simulink model "model_constInput_IPC"  (R2021b)
settings: Solver=ode4  StartTime=0.0  StopTime=simOpt.SLmaxTime  FixedStep=simOpt.SLsmplTime  RelTol=1e-3
values from neighbouring files (symbols this model uses):
  simOpt = simOptTmpl    [doSingleSim.m]    (also in doSingleSimVal.m)
  SLin = struct()    [doSingleSim.m]    (also in doSingleSimVal.m)
undefined symbols (not defined in the file or in its folder): DiscIntNeverNeededParam, Parameter, rpm2radDs, strmatch
libraries: simulink x14, dspstat3 x7, cstblocks x6, slpidlib x1
settings Model: Creator=Hazim Namik  LastModifiedBy=Manuel
settings SolverCC: AlgebraicLoopSolver=LineSearch
settings DataIOCC: LimitDataPoints=on  SaveFormat=Array  SaveOutput=off  SignalLogging=off  SaveTime=off  SignalLoggingName=sigsOut
settings OptimizationCC: BlockReduction=off  BooleanDataType=off  LifeSpan=inf
settings DebuggingCC: SaveWithParameterizedLinksMsg=none  UnderspecifiedInitializationDetection=Classic  MergeDetectMultiDrivingBlocksExec=none  AllowSymbolicDim=off  PregeneratedLibrarySubsystemCodeDiagnostic=none  SFUnexpectedBacktrackingDiag=warning  SFNoUnconditionalDefaultTransitionDiag=warning  SFExecutionAtInitializationDiag=none  SFMachineParentedDataDiag=warning  ArithmeticOperatorsInVariantConditions=warning
settings HardwareCC: ProdBitPerPointer=32  ProdBitPerSizeT=32  ProdBitPerPtrDiffT=32  ProdLargestAtomicFloat=None  ProdIntDivRoundTo=Undefined  ProdEndianess=Unspecified  ProdWordSize=32  ProdHWDeviceType=32-bit Generic  TargetBitPerPointer=64  TargetBitPerSizeT=64  TargetBitPerPtrDiffT=64  TargetLongLongMode=on  TargetIntDivRoundTo=Zero  TargetEndianess=LittleEndian  TargetWordSize=64  TargetHWDeviceType=MATLAB Host  ProdEqTarget=off
settings ModelReferenceCC: PropagateSignalLabelsOutOfModel=off
settings SFSimCC: SimUseLocalCustomCode=off  CustomCodeUndefinedFunction=UseInterfaceOnly
settings RTWCC: RTWUseLocalCustomCode=off
settings CodeAppCC: StateflowObjectComments=on
settings GRTTargetCC: TargetLangStandard=C89/C90 (ANSI)
settings ConfigComp: CovMetricSettings=dw  CovSaveCumulativeToWorkspaceVar=on  CovSaveSingleToWorkspaceVar=on  CovExternalEMLEnable=off  CovSFcnEnable=off

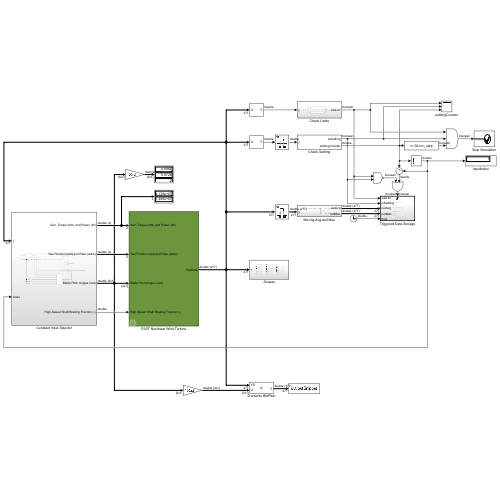
[thumbnail: Simulink's stored preview of the top-level diagram]
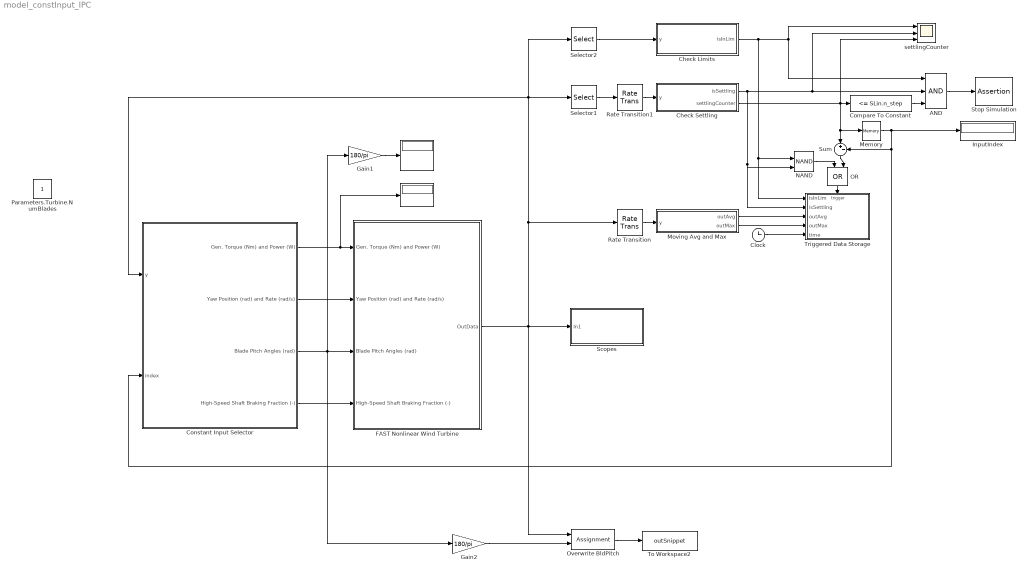
== system model_constInput_IPC ==
  " " : Display
  "  " : Display
  AND : Logic  Inputs=3  IconShape=distinctive  AllPortsSameDT=off  OutDataTypeStr=boolean
  Check Limits : Subsystem
  Check Settling : Subsystem
  Clock : Clock
  Compare To Constant : simulink/Logic and Bit Operations/Compare To Constant  relop=<=  const=SLin.n_step  OutDataTypeStr=boolean
  Constant Input Selector : Subsystem
  FAST Nonlinear Wind Turbine : Subsystem  mask(FAST Nonlinear Wind Turbine){}
      mask help: This block contains the FAST S-Function.
      mask init:
      | clear FAST_SFunc
  Gain1 : Gain  Gain=180/pi
  Gain2 : Gain  Gain=180/pi
  InputIndex : Display
  Memory : Memory  InitialCondition=1
  Moving Avg and Max : Subsystem
  NAND : Logic  Operator=NAND  IconShape=distinctive  AllPortsSameDT=off  OutDataTypeStr=boolean
  OR : Logic  Operator=OR  IconShape=distinctive  AllPortsSameDT=off  OutDataTypeStr=boolean
  Overwrite BldPitch : Assignment  DiagnosticForDimensions=Warning  IndexOptions=Index vector (dialog)  Indices=[simOpt.idx.y.BldPitch1 simOpt.idx.y.BldPitch2 simOpt.idx.y.BldPitch3]  OutputSizes=1
  Rate Transition : RateTransition
  Rate Transition1 : RateTransition
  Scopes : Subsystem
  Selector1 : Selector  InputPortWidth=simOpt.n_out  IndexOptions=Index vector (dialog)  Indices=simOpt.idx.y.settling  OutputSizes=1
  Selector2 : Selector  InputPortWidth=simOpt.n_out  IndexOptions=Index vector (dialog)  Indices=simOpt.idx.y.limCheck  OutputSizes=1
  Stop Simulation : Assertion  AssertionFailFcn=set_param(bdroot,'SimulationCommand','stop')  StopWhenAssertionFail=off
  Sum : Sum  Inputs=|+-
  To Workspace2 : ToWorkspace  VariableName=outSnippet  SampleTime=-1
      settings: MaxDataPoints=simOpt.settlingMovAvgWindowLength*5
  "Triggered Data Storage " : Subsystem  TreatAsAtomicUnit=on
  settlingCounter : Scope  NumInputPorts=3
  Parameters.Turbine.NumBlades : Constant  IOType=siggen
  wires:
  Selector1/1 -> Rate Transition1/1
  Rate Transition/1 -> Moving Avg and Max/1(y)
  Rate Transition1/1 -> Check Settling/1(y)
  Selector2/1 -> Check Limits/1(y)
  Check Limits/1(isInLim) -> NAND/1, "Triggered Data Storage "/1(isInLim), settlingCounter/1, AND/1
  Check Settling/1(isSettling) -> NAND/2, "Triggered Data Storage "/2(isSettling), settlingCounter/2, AND/2
  Moving Avg and Max/1(outAvg) -> "Triggered Data Storage "/3(outAvg)
  AND/1 -> Stop Simulation/1
  Compare To Constant/1 -> AND/3
  Clock/1 -> "Triggered Data Storage "/5(time)
  Check Settling/2(settlingCounter) -> Sum/1, Memory/1, settlingCounter/3, Compare To Constant/1
  Memory/1 -> InputIndex/1, Constant Input Selector/2(index), Sum/2
  Constant Input Selector/1(Gen. Torque (Nm) and Power (W)) -> "  "/1, FAST Nonlinear Wind Turbine/1(Gen. Torque (Nm) and Power (W))
  Constant Input Selector/2(Yaw Position (rad) and Rate (rad/s)) -> FAST Nonlinear Wind Turbine/2(Yaw Position (rad) and Rate (rad/s))
  Constant Input Selector/3(Blade Pitch Angles (rad)) -> Gain2/1, Gain1/1, FAST Nonlinear Wind Turbine/3(Blade Pitch Angles (rad))
  Constant Input Selector/4(High-Speed Shaft Braking Fraction (-)) -> FAST Nonlinear Wind Turbine/4(High-Speed Shaft Braking Fraction (-))
  Gain1/1 -> " "/1
  OR/1 -> "Triggered Data Storage "/Trigger
  Sum/1 -> OR/2
  NAND/1 -> OR/1
  FAST Nonlinear Wind Turbine/1(OutData) -> Overwrite BldPitch/1, Constant Input Selector/1(y), Selector1/1, Selector2/1, Rate Transition/1, Scopes/1(In1)
  Moving Avg and Max/2(outMax) -> "Triggered Data Storage "/4(outMax)
  Overwrite BldPitch/1 -> To Workspace2/1
  Gain2/1 -> Overwrite BldPitch/2

== system model_constInput_IPC/Check Limits ==
  y : Inport
  Compare To Constant : simulink/Logic and Bit Operations/Compare To Constant  relop=<=  const=simOpt.limCheckLowerBound  OutDataTypeStr=boolean
  Compare To Constant1 : simulink/Logic and Bit Operations/Compare To Constant  relop=>=  const=simOpt.limCheckUpperBound  OutDataTypeStr=boolean
  OR : Logic  Operator=NOR  IconShape=distinctive  AllPortsSameDT=off  OutDataTypeStr=boolean
  isInLim : Outport
  wires:
  y/1 -> Compare To Constant1/1, Compare To Constant/1
  OR/1 -> isInLim/1
  Compare To Constant1/1 -> OR/2
  Compare To Constant/1 -> OR/1

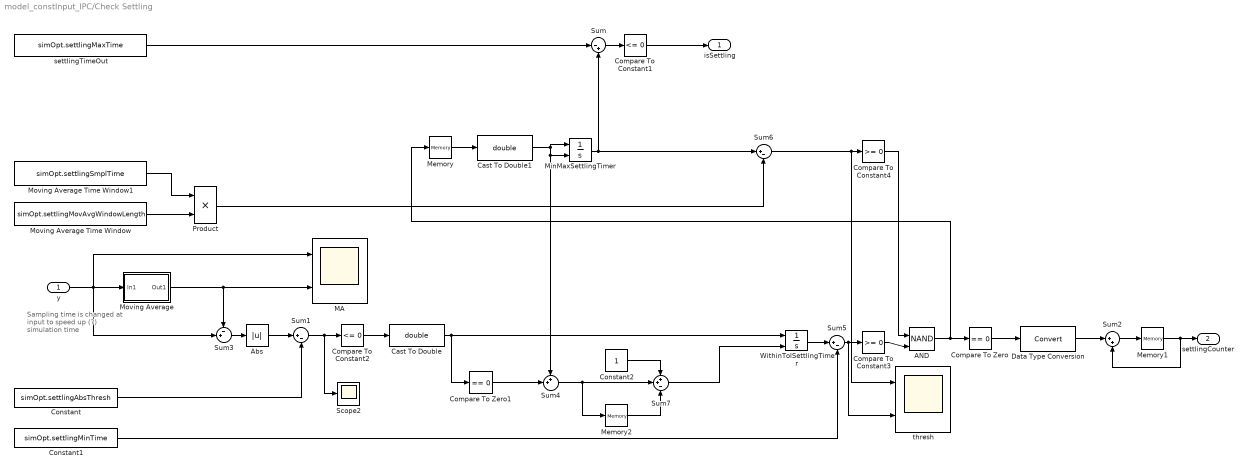
== system model_constInput_IPC/Check Settling ==
  note: Sampling time is changed at input
      | to speed up (?) simulation time
  y : Inport  SampleTime=simOpt.settlingSmplTime
  AND : Logic  Operator=NAND  IconShape=distinctive  AllPortsSameDT=off  OutDataTypeStr=boolean
  Abs : Abs
  Cast To Double : DataTypeConversion  OutDataTypeStr=double
  Cast To Double1 : DataTypeConversion  OutDataTypeStr=double
  Compare To Constant1 : simulink/Logic and Bit Operations/Compare To Constant  relop=<=  const=0  OutDataTypeStr=boolean
  Compare To Constant2 : simulink/Logic and Bit Operations/Compare To Constant  relop=<=  const=0  OutDataTypeStr=boolean
  Compare To Constant3 : simulink/Logic and Bit Operations/Compare To Constant  relop=>=  const=0  OutDataTypeStr=boolean
  Compare To Constant4 : simulink/Logic and Bit Operations/Compare To Constant  relop=>=  const=0  OutDataTypeStr=boolean
  Compare To Zero : simulink/Logic and Bit Operations/Compare To Zero  relop===  OutDataTypeStr=boolean
  Compare To Zero1 : simulink/Logic and Bit Operations/Compare To Zero  relop===  OutDataTypeStr=boolean
  Constant : Constant  Value=simOpt.settlingAbsThresh
  Constant1 : Constant  Value=simOpt.settlingMinTime
  Constant2 : Constant
  Data Type Conversion : DataTypeConversion
  MA : Scope  NumInputPorts=2
  Memory : Memory  InitialCondition=true
  Memory1 : Memory  InitialCondition=1  InheritSampleTime=on
  Memory2 : Memory  InitialCondition=1  InheritSampleTime=on
  MinMaxSettlingTimer : Integrator  ExternalReset=falling  LimitOutput=on  UpperSaturationLimit=max(simOpt.settlingMovAvgWindowLength*simOpt.settlingSmplTime,simOpt.settlingMaxTime)*1.01
  Moving Average : Subsystem
  Moving Average Time Window : Constant  Value=simOpt.settlingMovAvgWindowLength
  Moving Average Time Window1 : Constant  Value=simOpt.settlingSmplTime
  Product : Product
  Scope2 : Scope
  Sum : Sum  Inputs=|-+
  Sum1 : Sum  Inputs=|+-
  Sum2 : Sum  Inputs=|++
  Sum3 : Sum  Inputs=-+|
  Sum4 : Sum  Inputs=++|
  Sum5 : Sum  Inputs=|+-
  Sum6 : Sum  Inputs=|+-
  Sum7 : Sum  Inputs=++-
  WithinTolSettlingTimer : Integrator  ExternalReset=falling  LimitOutput=on  UpperSaturationLimit=simOpt.settlingMinTime
  settlingTimeOut : Constant  Value=simOpt.settlingMaxTime
  thresh : Scope  NumInputPorts=2
  isSettling : Outport
  settlingCounter : Outport  Port=2
  wires:
  AND/1 -> Compare To Zero/1, Memory/1
  MinMaxSettlingTimer/1 -> Sum6/1, Sum/2
  Sum6/1 -> thresh/1, Compare To Constant4/1
  Sum1/1 -> Scope2/1, Compare To Constant2/1
  WithinTolSettlingTimer/1 -> Sum5/1
  y/1 -> MA/1, Moving Average/1(In1), Sum3/2
  Abs/1 -> Sum1/1
  Sum3/1 -> Abs/1
  Sum5/1 -> thresh/2, Compare To Constant3/1
  Moving Average Time Window/1 -> Product/2
  Compare To Constant2/1 -> Cast To Double/1
  Constant/1 -> Sum1/2
  Constant1/1 -> Sum5/2
  Compare To Constant3/1 -> AND/2
  Compare To Constant4/1 -> AND/1
  Memory/1 -> Cast To Double1/1
  Cast To Double1/1 -> Sum4/1, MinMaxSettlingTimer/2, MinMaxSettlingTimer/1
  Moving Average/1(Out1) -> Sum3/1, MA/2
  settlingTimeOut/1 -> Sum/1
  Sum/1 -> Compare To Constant1/1
  Compare To Constant1/1 -> isSettling/1
  Memory1/1 -> settlingCounter/1, Sum2/2
  Sum2/1 -> Memory1/1
  Compare To Zero/1 -> Data Type Conversion/1
  Data Type Conversion/1 -> Sum2/1
  Moving Average Time Window1/1 -> Product/1
  Product/1 -> Sum6/2
  Sum7/1 -> WithinTolSettlingTimer/2
  Compare To Zero1/1 -> Sum4/2
  Cast To Double/1 -> WithinTolSettlingTimer/1, Compare To Zero1/1
  Sum4/1 -> Sum7/2, Memory2/1
  Memory2/1 -> Sum7/3
  Constant2/1 -> Sum7/1

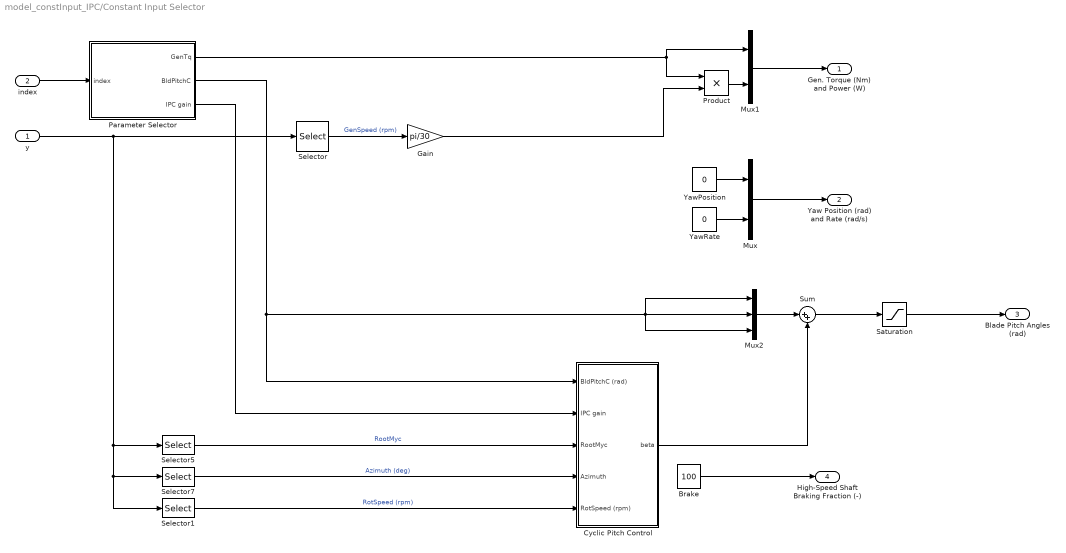
== system model_constInput_IPC/Constant Input Selector ==
  y : Inport
  index : Inport  Port=2
  Brake : Constant  Value=100
  Cyclic Pitch Control : Subsystem
  Gain : Gain  Gain=pi/30
  Mux : Mux  Inputs=2
  Mux1 : Mux  Inputs=2
  Mux2 : Mux  Inputs=3
  Parameter Selector : Subsystem
  Product : Product
  Saturation : Saturate  UpperLimit=inf  LowerLimit=deg2rad(simOpt.BldPitch_min)
  Selector : Selector  InputPortWidth=simOpt.n_out  IndexOptions=Index vector (dialog)  Indices=simOpt.idx.y.GenSpeed  OutputSizes=1
  Selector1 : Selector  InputPortWidth=simOpt.n_out  IndexOptions=Index vector (dialog)  Indices=simOpt.idx.y.RotSpeed  OutputSizes=1
  Selector5 : Selector  InputPortWidth=simOpt.n_out  IndexOptions=Index vector (dialog)  Indices=[simOpt.idx.y.RootMyc1 simOpt.idx.y.RootMyc2 simOpt.idx.y.RootMyc3]  OutputSizes=1
  Selector7 : Selector  InputPortWidth=simOpt.n_out  IndexOptions=Index vector (dialog)  Indices=simOpt.idx.y.Azimuth  OutputSizes=1
  Sum : Sum  Inputs=|++
  YawPosition : Constant  Value=0
  YawRate : Constant  Value=0
  Gen. Torque (Nm) and Power (W) : Outport
  Yaw Position (rad) and Rate (rad/s) : Outport  Port=2
  Blade Pitch Angles (rad) : Outport  Port=3
  High-Speed Shaft Braking Fraction (-) : Outport  Port=4
  wires:
  YawRate/1 -> Mux/2
  index/1 -> Parameter Selector/1(index)
  YawPosition/1 -> Mux/1
  Product/1 -> Mux1/2
  Brake/1 -> High-Speed Shaft Braking Fraction (-)/1
  Mux1/1 -> Gen. Torque (Nm) and Power (W)/1
  Mux/1 -> Yaw Position (rad) and Rate (rad/s)/1
  Gain/1 -> Product/2
  Parameter Selector/2(BldPitchC) -> Cyclic Pitch Control/1(BldPitchC (rad)), Mux2/1, Mux2/3, Mux2/2
  Mux2/1 -> Sum/1
  y/1 -> Selector/1, Selector1/1, Selector7/1, Selector5/1
  Selector/1 -> Gain/1  "GenSpeed (rpm)"
  Selector5/1 -> Cyclic Pitch Control/3(RootMyc)  "RootMyc"
  Selector7/1 -> Cyclic Pitch Control/4(Azimuth)  "Azimuth (deg)"
  Cyclic Pitch Control/1(beta) -> Sum/2
  Parameter Selector/3(IPC gain) -> Cyclic Pitch Control/2(IPC gain)
  Parameter Selector/1(GenTq) -> Mux1/1, Product/1
  Selector1/1 -> Cyclic Pitch Control/5(RotSpeed (rpm))  "RotSpeed (rpm)"
  Sum/1 -> Saturation/1
  Saturation/1 -> Blade Pitch Angles (rad)/1

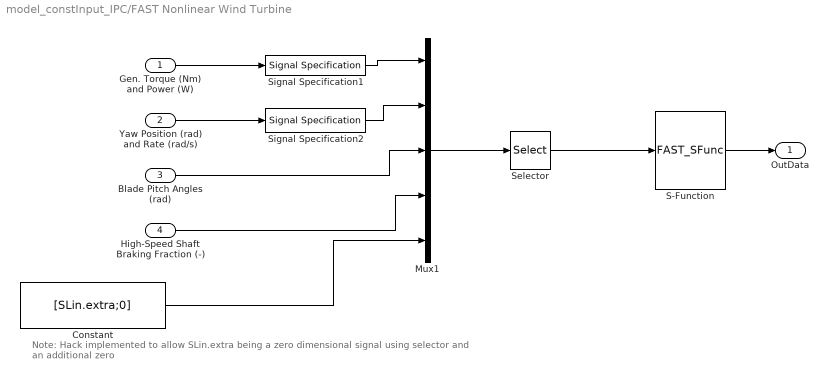
== system model_constInput_IPC/FAST Nonlinear Wind Turbine ==
  note: Note: Hack implemented to allow SLin.extra being a zero dimensional signal using selector and an additional zero
  Gen. Torque (Nm) and Power (W) : Inport
  Yaw Position (rad) and Rate (rad/s) : Inport  Port=2
  Blade Pitch Angles (rad) : Inport  Port=3
  High-Speed Shaft Braking Fraction (-) : Inport  Port=4
  Constant : Constant  Value=[SLin.extra;0]
  Mux1 : Mux  Inputs=5
  S-Function : S-Function  FunctionName=FAST_SFunc  Parameters=simOpt.FSTnewInputFile, simOpt.SLmaxTime, 0  SFunctionDeploymentMode=off  EnableBusSupport=off
  Selector : Selector  InputPortWidth=9+numel(SLin.extra)  IndexOptions=Index vector (dialog)  Indices=1:(8+numel(SLin.extra))  OutputSizes=1
  Signal Specification1 : SignalSpecification  OutDataTypeStr=double  Dimensions=2
  Signal Specification2 : SignalSpecification  OutDataTypeStr=double  Dimensions=2
  OutData : Outport  VectorParamsAs1DForOutWhenUnconnected=off
  wires:
  Gen. Torque (Nm) and Power (W)/1 -> Signal Specification1/1
  S-Function/1 -> OutData/1
  Mux1/1 -> Selector/1
  Blade Pitch Angles (rad)/1 -> Mux1/3
  Yaw Position (rad) and Rate (rad/s)/1 -> Signal Specification2/1
  Signal Specification1/1 -> Mux1/1
  Signal Specification2/1 -> Mux1/2
  High-Speed Shaft Braking Fraction (-)/1 -> Mux1/4
  Constant/1 -> Mux1/5
  Selector/1 -> S-Function/1

== system model_constInput_IPC/Moving Avg and Max ==
  note: Sampling time is changed at input
      | to speed up (?) simulation time
  y : Inport  SampleTime=simOpt.settlingSmplTime
  Moving Maximum : dspstat3/Moving Maximum  SpecifyWindowLength=on  WindowLength=simOpt.settlingMovAvgWindowLength  SimulateUsing=Interpreted execution
      settings: SourceProductBaseCode=DS
  Moving Average : dspstat3/Moving Average  Method=Sliding window  ForgettingFactorPort=off  SpecifyWindowLength=on  WindowLength=simOpt.settlingMovAvgWindowLength  ForgettingFactor=0.99  SimulateUsing=Interpreted execution
  Reshape : Reshape  OutputDimensionality=Row vector (2-D)
  Reshape1 : Reshape
  Reshape2 : Reshape
  outAvg : Outport
  outMax : Outport  Port=2
  wires:
  y/1 -> Reshape/1
  Moving Average/1 -> Reshape1/1
  Reshape/1 -> Moving Maximum/1, Moving Average/1
  Reshape1/1 -> outAvg/1
  Reshape2/1 -> outMax/1
  Moving Maximum/1 -> Reshape2/1

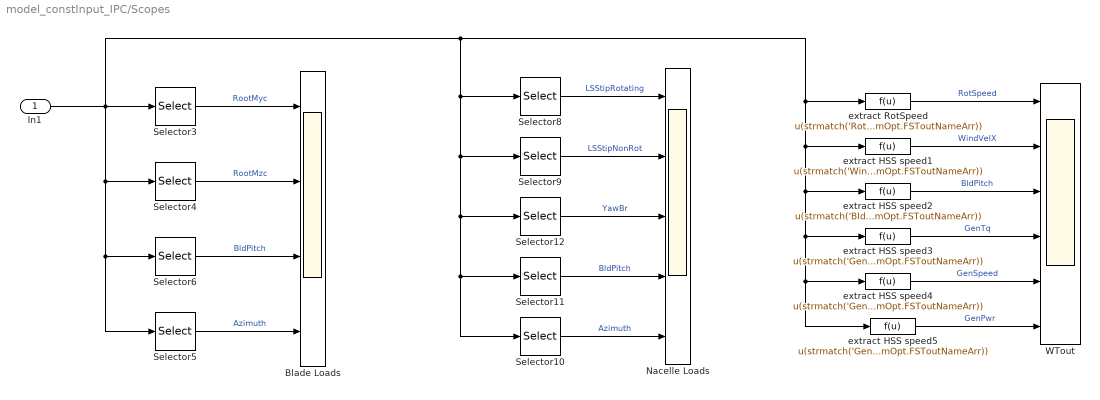
== system model_constInput_IPC/Scopes ==
  In1 : Inport
  Blade Loads : Scope  NumInputPorts=4
  Nacelle Loads : Scope  NumInputPorts=5
  Selector10 : Selector  InputPortWidth=simOpt.n_out  IndexOptions=Index vector (dialog)  Indices=[simOpt.idx.y.Azimuth]  OutputSizes=1
  Selector11 : Selector  InputPortWidth=simOpt.n_out  IndexOptions=Index vector (dialog)  Indices=[simOpt.idx.y.BldPitch1 simOpt.idx.y.BldPitch2 simOpt.idx.y.BldPitch3]  OutputSizes=1
  Selector12 : Selector  InputPortWidth=simOpt.n_out  IndexOptions=Index vector (dialog)  Indices=[simOpt.idx.y.YawBrMyp simOpt.idx.y.YawBrMzp]  OutputSizes=1
  Selector3 : Selector  InputPortWidth=simOpt.n_out  IndexOptions=Index vector (dialog)  Indices=[simOpt.idx.y.RootMyc1 simOpt.idx.y.RootMyc2 simOpt.idx.y.RootMyc3]  OutputSizes=1
  Selector4 : Selector  InputPortWidth=simOpt.n_out  IndexOptions=Index vector (dialog)  Indices=[simOpt.idx.y.RootMzc1 simOpt.idx.y.RootMzc2 simOpt.idx.y.RootMzc3]  OutputSizes=1
  Selector5 : Selector  InputPortWidth=simOpt.n_out  IndexOptions=Index vector (dialog)  Indices=[simOpt.idx.y.Azimuth]  OutputSizes=1
  Selector6 : Selector  InputPortWidth=simOpt.n_out  IndexOptions=Index vector (dialog)  Indices=[simOpt.idx.y.BldPitch1 simOpt.idx.y.BldPitch2 simOpt.idx.y.BldPitch3]  OutputSizes=1
  Selector8 : Selector  InputPortWidth=simOpt.n_out  IndexOptions=Index vector (dialog)  Indices=[simOpt.idx.y.LSSTipMya simOpt.idx.y.LSSTipMza]  OutputSizes=1
  Selector9 : Selector  InputPortWidth=simOpt.n_out  IndexOptions=Index vector (dialog)  Indices=[simOpt.idx.y.LSSTipMys simOpt.idx.y.LSSTipMzs]  OutputSizes=1
  WTout : Scope  NumInputPorts=6
  extract HSS speed1 : Fcn  Expr=u(strmatch('Wind1VelX',simOpt.FSToutNameArr))
  extract HSS speed2 : Fcn  Expr=u(strmatch('BldPitch1',simOpt.FSToutNameArr))
  extract HSS speed3 : Fcn  Expr=u(strmatch('GenTq',simOpt.FSToutNameArr))
  extract HSS speed4 : Fcn  Expr=u(strmatch('GenSpeed',simOpt.FSToutNameArr))
  extract HSS speed5 : Fcn  Expr=u(strmatch('GenPwr',simOpt.FSToutNameArr))
  extract RotSpeed : Fcn  Expr=u(strmatch('RotSpeed',simOpt.FSToutNameArr))
  wires:
  In1/1 -> Selector5/1, Selector6/1, Selector4/1, Selector10/1, Selector11/1, Selector12/1, Selector9/1, Selector8/1, extract RotSpeed/1, extract HSS speed1/1, extract HSS speed3/1, extract HSS speed4/1, extract HSS speed5/1, extract HSS speed2/1, Selector3/1
  Selector6/1 -> Blade Loads/3  "BldPitch"
  Selector9/1 -> Nacelle Loads/2  "LSStipNonRot"
  extract HSS speed5/1 -> WTout/6  "GenPwr"
  Selector3/1 -> Blade Loads/1  "RootMyc"
  Selector8/1 -> Nacelle Loads/1  "LSStipRotating"
  Selector11/1 -> Nacelle Loads/4  "BldPitch"
  extract HSS speed2/1 -> WTout/3  "BldPitch"
  extract RotSpeed/1 -> WTout/1  "RotSpeed"
  Selector5/1 -> Blade Loads/4  "Azimuth"
  Selector12/1 -> Nacelle Loads/3  "YawBr"
  extract HSS speed4/1 -> WTout/5  "GenSpeed"
  extract HSS speed1/1 -> WTout/2  "WindVelX"
  Selector10/1 -> Nacelle Loads/5  "Azimuth"
  extract HSS speed3/1 -> WTout/4  "GenTq"
  Selector4/1 -> Blade Loads/2  "RootMzc"

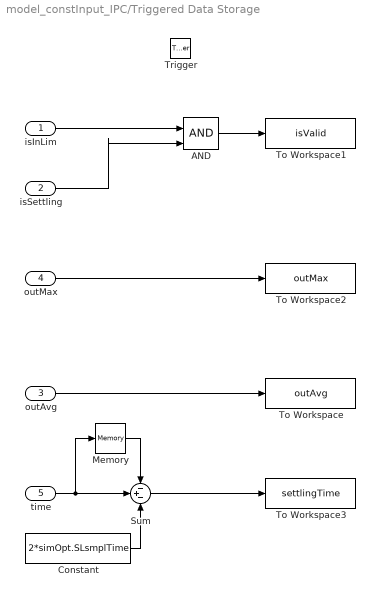
== system model_constInput_IPC/Triggered Data Storage  ==
  isInLim : Inport
  isSettling : Inport  Port=2
  outAvg : Inport  Port=3
  outMax : Inport  Port=4
  time : Inport  Port=5
  Trigger : TriggerPort  VariantControl=(inherit)
  AND : Logic  IconShape=distinctive  AllPortsSameDT=off  OutDataTypeStr=boolean
  Constant : Constant  Value=2*simOpt.SLsmplTime
  Memory : Memory  InheritSampleTime=on
  Sum : Sum  Inputs=-+-
  To Workspace : ToWorkspace  VariableName=outAvg  SampleTime=-1
  To Workspace1 : ToWorkspace  VariableName=isValid  SampleTime=-1
  To Workspace2 : ToWorkspace  VariableName=outMax  SampleTime=-1
  To Workspace3 : ToWorkspace  VariableName=settlingTime  SampleTime=-1
  wires:
  outAvg/1 -> To Workspace/1
  isInLim/1 -> AND/1
  isSettling/1 -> AND/2
  Sum/1 -> To Workspace3/1
  time/1 -> Sum/2, Memory/1
  AND/1 -> To Workspace1/1
  Constant/1 -> Sum/3
  Memory/1 -> Sum/1
  outMax/1 -> To Workspace2/1

== system model_constInput_IPC/Check Settling/Moving Average ==
  In1 : Inport
  Moving Average : dspstat3/Moving Average  Method=Sliding window  ForgettingFactorPort=off  SpecifyWindowLength=on  WindowLength=simOpt.settlingMovAvgWindowLength  ForgettingFactor=0.99  SimulateUsing=Interpreted execution
  Reshape : Reshape  OutputDimensionality=Row vector (2-D)
  Reshape1 : Reshape
  Out1 : Outport
  wires:
  Moving Average/1 -> Reshape1/1
  Reshape1/1 -> Out1/1
  Reshape/1 -> Moving Average/1
  In1/1 -> Reshape/1

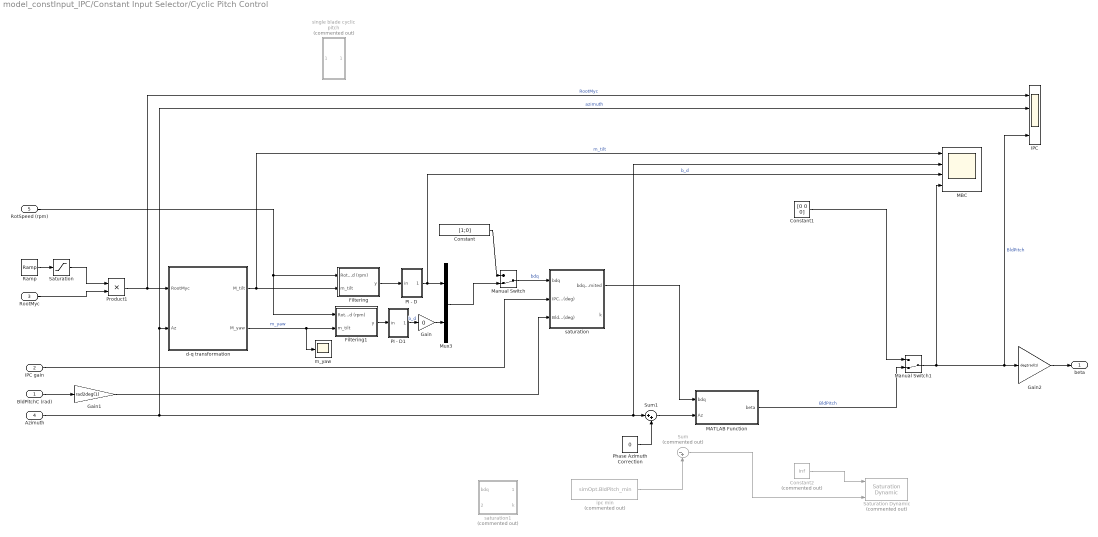
== system model_constInput_IPC/Constant Input Selector/Cyclic Pitch Control ==
  BldPitchC (rad) : Inport
  IPC gain : Inport  Port=2
  RootMyc : Inport  Port=3
  Azimuth : Inport  Port=4
  RotSpeed (rpm) : Inport  Port=5
  Constant : Constant  Value=[1;0]
  Constant1 : Constant  Value=[0 0 0]
  Constant2 : Constant  Commented=on  Value=inf
  Filtering : Subsystem
  Filtering1 : Subsystem
  Gain : Gain  Gain=0
  Gain1 : Gain  Gain=rad2deg(1)
  Gain2 : Gain  Gain=deg2rad(1)
  IPC : Scope  NumInputPorts=4
  MATLAB Function : MATLAB Function  TreatAsAtomicUnit=on
  MBC : Scope  NumInputPorts=4
  Manual Switch : ManualSwitch  CurrentSetting=0
  Manual Switch1 : ManualSwitch  CurrentSetting=0
  Mux3 : Mux  Inputs=2
  PI - D : Subsystem
  PI - D1 : Subsystem
  Phase Azimuth Correction : Constant  Value=0
  Product1 : Product
  Ramp : simulink/Sources/Ramp  slope=1  start=0  InitialOutput=0
  Saturation : Saturate  UpperLimit=1  LowerLimit=0
  Saturation Dynamic : simulink/Discontinuities/Saturation Dynamic  Commented=on  OutMin=[]  OutMax=[]  OutDataTypeStr=Inherit: Same as second input  OutDataType=fixdt(1, 16)  OutScaling=2^-10  DoSatur=off
  Sum : Sum  Commented=on  Inputs=|-+
  Sum1 : Sum  Inputs=|++
  d-q transformation : MATLAB Function  TreatAsAtomicUnit=on
  ipc min : Constant  Commented=on  Value=simOpt.BldPitch_min
  m_yaw : Scope
  saturation : Subsystem
  saturation1 : Subsystem  Commented=on
  single blade cyclic pitch : Subsystem  Commented=on
  beta : Outport
  wires:
  Azimuth/1 -> IPC/2, d-q transformation/2(Az), MBC/2, Sum1/1  "azimuth"
  d-q transformation/2(M_yaw) -> Filtering1/2(m_tilt), m_yaw/1  "m_yaw"
  Product1/1 -> IPC/1, d-q transformation/1(RootMyc)  "RootMyc"
  Filtering1/1(y) -> PI - D1/1(in)
  Constant/1 -> Manual Switch/1
  d-q transformation/1(M_tilt) -> Filtering/2(m_tilt), MBC/1  "m_tilt"
  Mux3/1 -> Manual Switch/2
  Manual Switch1/1 -> Gain2/1, IPC/4, MBC/4  "BldPitch"
  Constant1/1 -> Manual Switch1/1
  IPC gain/1 -> saturation/2(IPCbldPitch_abs_max (deg))
  Manual Switch/1 -> saturation/1(bdq)  "bdq"
  Filtering/1(y) -> PI - D/1(in)
  RotSpeed (rpm)/1 -> Filtering1/1(RotSpeed (rpm)), Filtering/1(RotSpeed (rpm))
  PI - D/1(out) -> MBC/3, Mux3/1  "b_d"
  Sum1/1 -> MATLAB Function/2(Az)
  Phase Azimuth Correction/1 -> Sum1/2
  PI - D1/1(out) -> Gain/1  "b_d"
  Gain/1 -> Mux3/2
  RootMyc/1 -> Product1/2
  Saturation/1 -> Product1/1
  Ramp/1 -> Saturation/1
  saturation/1(bdq_limited) -> MATLAB Function/1(bdq)
  BldPitchC (rad)/1 -> Gain1/1
  Gain1/1 -> saturation/3(BldPitchC (deg))
  MATLAB Function/1(beta) -> Manual Switch1/2  "BldPitch"
  ipc min/1 -> Sum/2
  Sum/1 -> Saturation Dynamic/3
  Constant2/1 -> Saturation Dynamic/1
  Gain2/1 -> beta/1

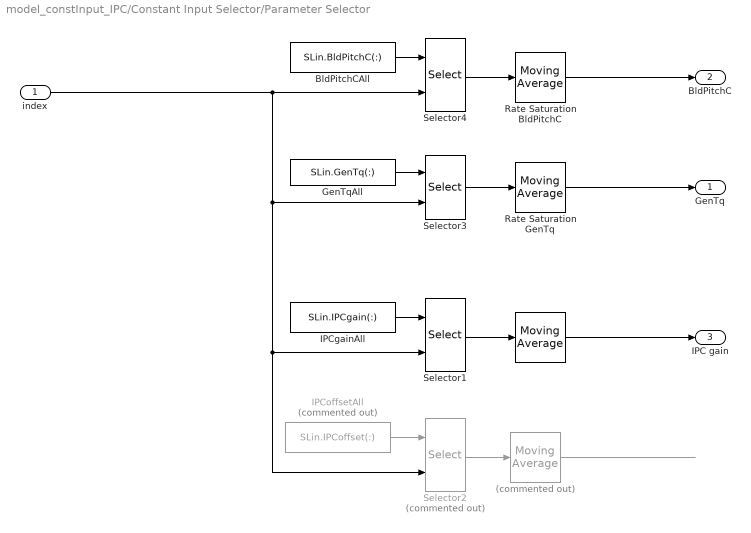
== system model_constInput_IPC/Constant Input Selector/Parameter Selector ==
  index : Inport
  " " : dspstat3/Moving Average  Method=Sliding window  ForgettingFactorPort=off  SpecifyWindowLength=on  WindowLength=8  ForgettingFactor=0.99  SimulateUsing=Interpreted execution
  "  " : dspstat3/Moving Average  Commented=on  Method=Sliding window  ForgettingFactorPort=off  SpecifyWindowLength=on  WindowLength=8  ForgettingFactor=0.99  SimulateUsing=Interpreted execution
  BldPitchCAll : Constant  Value=SLin.BldPitchC(:)
  GenTqAll : Constant  Value=SLin.GenTq(:)
  IPCgainAll : Constant  Value=SLin.IPCgain(:)
  IPCoffsetAll : Constant  Commented=on  Value=SLin.IPCoffset(:)
  Rate Saturation BldPitchC : dspstat3/Moving Average  Method=Sliding window  ForgettingFactorPort=off  SpecifyWindowLength=on  WindowLength=8  ForgettingFactor=0.99  SimulateUsing=Interpreted execution
  Rate Saturation GenTq : dspstat3/Moving Average  Method=Sliding window  ForgettingFactorPort=off  SpecifyWindowLength=on  WindowLength=8  ForgettingFactor=0.99  SimulateUsing=Interpreted execution
  Selector1 : Selector  InputPortWidth=SLin.n_step  IndexOptions=Index vector (port)  Indices=simOpt.i_outRotSpeed  OutputSizes=1
  Selector2 : Selector  Commented=on  InputPortWidth=SLin.n_step  IndexOptions=Index vector (port)  Indices=simOpt.i_outRotSpeed  OutputSizes=1
  Selector3 : Selector  InputPortWidth=SLin.n_step  IndexOptions=Index vector (port)  Indices=simOpt.i_outRotSpeed  OutputSizes=1
  Selector4 : Selector  InputPortWidth=SLin.n_step  IndexOptions=Index vector (port)  Indices=simOpt.i_outRotSpeed  OutputSizes=1
  GenTq : Outport
  BldPitchC : Outport  Port=2
  IPC gain : Outport  Port=3
  wires:
  IPCgainAll/1 -> Selector1/1
  "  "/1 -> ?
  Selector1/1 -> " "/1
  " "/1 -> IPC gain/1
  Selector2/1 -> "  "/1
  IPCoffsetAll/1 -> Selector2/1
  GenTqAll/1 -> Selector3/1
  Selector3/1 -> Rate Saturation GenTq/1
  Rate Saturation GenTq/1 -> GenTq/1
  index/1 -> Selector3/2, Selector2/2, Selector1/2, Selector4/2
  BldPitchCAll/1 -> Selector4/1
  Selector4/1 -> Rate Saturation BldPitchC/1
  Rate Saturation BldPitchC/1 -> BldPitchC/1

== system model_constInput_IPC/Constant Input Selector/Cyclic Pitch Control/Filtering ==
  RotSpeed (rpm) : Inport
  m_tilt : Inport  Port=2
  Gain1 : Gain  Gain=rpm2radDs
  Moving 3P Notch : Subsystem
  Moving 6P Notch : Subsystem  Commented=on
  Moving Low Pass : Subsystem
  y : Outport
  wires:
  Moving 3P Notch/1(y) -> Moving Low Pass/1(u)
  Gain1/1 -> Moving Low Pass/2(RotSpeed (rad/s)), Moving 3P Notch/2(RotSpeed (rad/s))
  m_tilt/1 -> Moving 3P Notch/1(u)
  RotSpeed (rpm)/1 -> Gain1/1
  Moving Low Pass/1(y) -> y/1

== system model_constInput_IPC/Constant Input Selector/Cyclic Pitch Control/Filtering1 ==
  RotSpeed (rpm) : Inport
  m_tilt : Inport  Port=2
  Gain1 : Gain  Gain=rpm2radDs
  Moving 3P Notch : Subsystem
  Moving 6P Notch : Subsystem  Commented=on
  Moving Low Pass : Subsystem
  y : Outport
  wires:
  Moving 3P Notch/1(y) -> Moving Low Pass/1(u)
  Gain1/1 -> Moving Low Pass/2(RotSpeed (rad/s)), Moving 3P Notch/2(RotSpeed (rad/s))
  m_tilt/1 -> Moving 3P Notch/1(u)
  RotSpeed (rpm)/1 -> Gain1/1
  Moving Low Pass/1(y) -> y/1

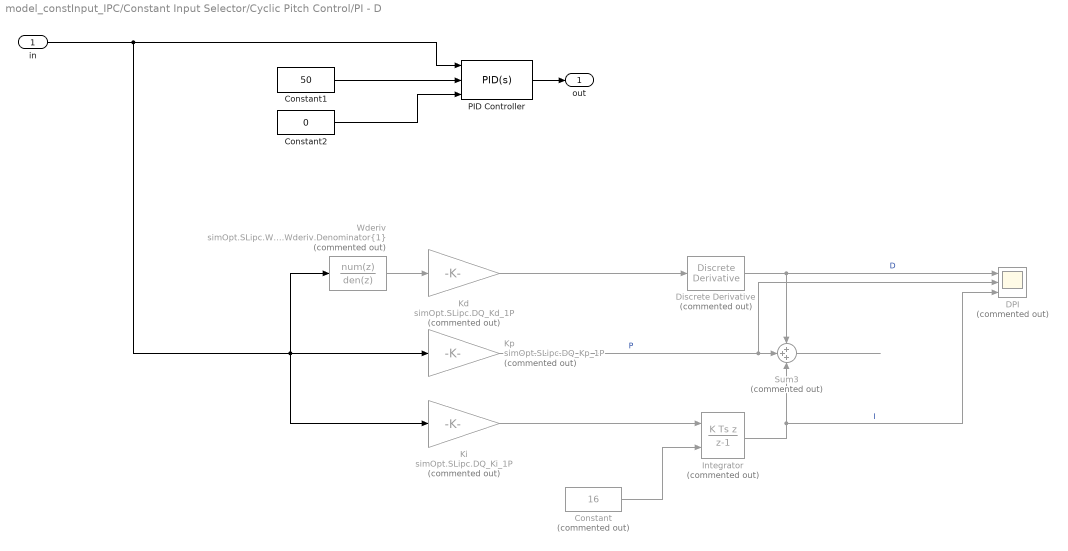
== system model_constInput_IPC/Constant Input Selector/Cyclic Pitch Control/PI - D ==
  in : Inport
  Constant : Constant  Commented=on  Value=16
  Constant1 : Constant  Value=50
  Constant2 : Constant  Value=0
  DPI : Scope  Commented=on  NumInputPorts=3
  Discrete Derivative : simulink/Discrete/Discrete Derivative  Commented=on  gainval=1.0  ICPrevScaledInput=0.0  OutMin=[]  OutMax=[]  OutDataType=fixdt(1, 16)  OutScaling=2^-10  DoSatur=off
  Integrator : DiscreteIntegrator  Commented=on  IntegratorMethod=Integration: Backward Euler  gainval=1  InitialConditionSource=external  SampleTime=-1  UpperSaturationLimit=1.570796/(.008068634/9.5492966)/(1./(1.+pi/2/.109997))  LowerSaturationLimit=0  ICPrevOutput=DiscIntNeverNeededParam  ICPrevScaledInput=DiscIntNeverNeededParam
  Kd : Gain  Commented=on  Gain=simOpt.SLipc.DQ_Kd_1P
  Ki : Gain  Commented=on  Gain=simOpt.SLipc.DQ_Ki_1P
  Kp : Gain  Commented=on  Gain=simOpt.SLipc.DQ_Kp_1P
  PID Controller : slpidlib/PID Controller  Controller=PID  Form=Parallel  TimeDomain=Continuous-time  UseExternalTs=off  SampleTime=-1  IntegratorMethod=Forward Euler  FilterMethod=Forward Euler  ControllerParametersSource=internal  P=simOpt.SLipc.DQ_Kp_1P  I=simOpt.SLipc.DQ_Ki_1P  D=simOpt.SLipc.DQ_Kd_1P  UseFilter=on  N=100  TunerSelectOption=Transfer Function Based (PID Tuner App)  InitialConditionSource=external  InitialConditionForIntegrator=0  InitialConditionForFilter=0  DifferentiatorICPrevScaledInput=0  ExternalReset=none  TrackingMode=off  Kt=1  LimitOutput=on  SatLimitsSource=internal  UpperSaturationLimit=90  LowerSaturationLimit=90  LinearizeAsGain=on  AntiWindupMode=clamping  Kb=1  POutMin=[]  POutMax=[]  IOutMin=[]  IOutMax=[]  DOutMin=[]  DOutMax=[]  NOutMin=[]  NOutMax=[]  SumOutMin=[]  SumOutMax=[]  SaturationOutMin=[]  SaturationOutMax=[]  PParamMin=[]  PParamMax=[]  IParamMin=[]  IParamMax=[]  DParamMin=[]  DParamMax=[]  NParamMin=[]  NParamMax=[]  KbParamMin=[]  KbParamMax=[]  KtParamMin=[]  KtParamMax=[]  KbOutMin=[]  KbOutMax=[]  KtOutMin=[]  KtOutMax=[]  IntegratorOutMin=[]  IntegratorOutMax=[]  FilterOutMin=[]  FilterOutMax=[]  SumI1OutMin=[]  SumI1OutMax=[]  SumI2OutMin=[]  SumI2OutMax=[]  SumI3OutMin=[]  SumI3OutMax=[]  SumI4OutMin=[]  SumI4OutMax=[]  SumDOutMin=[]  SumDOutMax=[]  DifferentiatorOutMin=[]  DifferentiatorOutMax=[]  FilterDiffOutCoefMin=[]  FilterDiffOutCoefMax=[]  ReciprocalOutMin=[]  ReciprocalOutMax=[]  SumDenOutMin=[]  SumDenOutMax=[]  SumNumOutMin=[]  SumNumOutMax=[]  DivideOutMin=[]  DivideOutMax=[]  UdiffTsProdOutMin=[]  UdiffTsProdOutMax=[]  NTsProdOutMin=[]  NTsProdOutMax=[]  UintegralTsProdOutMin=[]  UintegralTsProdOutMax=[]  UngainTsProdOutMin=[]  UngainTsProdOutMax=[]  IntegratorContinuousStateAttributes=''  IntegratorStateMustResolveToSignalObject=off  IntegratorRTWStateStorageClass=Auto  FilterContinuousStateAttributes=''  FilterStateMustResolveToSignalObject=off  FilterRTWStateStorageClass=Auto  ParallelPVariant=InternalParameters  IdealPVariant=Disabled  IVariant=InternalParameters  DVariant=InternalParameters  IntegratorVariant=Continuous  SatVariant=Enabled  AWVariant=ContClampingParallel  PCopyVariant=Disabled  TRVariant=Disabled  FdbkBlocksVariant=Forward  IdealPFdbkVariant=Disabled  SatFdbkVariant=Disabled  DerivativeFilterVariant=ContFilter  NVariant=InternalParameters  NCopyVariant=Disabled  FilterICVariant=ExternalICs  IntegratorICVariant=ExternalICs  ExternalResetVariant=Disabled  TRSumVariant=Passthrough  SumFdbkVariant=Disabled  SumVariant=Sum_PID  TsampFilterVariant=InternalTs  TsampNgainVariant=Passthrough  TsampIntegralVariant=Passthrough  ExternalSaturationOutDataTypeStr=Inherit: Same as second input
  Sum3 : Sum  Commented=on  Inputs=+++
  Wderiv : DiscreteFilter  Commented=on  Numerator=simOpt.SLipc.Wderiv.Numerator{1}  Denominator=simOpt.SLipc.Wderiv.Denominator{1}
  out : Outport  VectorParamsAs1DForOutWhenUnconnected=off
  wires:
  Wderiv/1 -> Kd/1
  Sum3/1 -> ?
  Kp/1 -> DPI/2, Sum3/2  "P"
  Discrete Derivative/1 -> Sum3/1, DPI/1  "D"
  Kd/1 -> Discrete Derivative/1
  in/1 -> Ki/1, Wderiv/1, Kp/1, PID Controller/1
  Integrator/1 -> DPI/3, Sum3/3  "I"
  Ki/1 -> Integrator/1
  Constant/1 -> Integrator/2
  PID Controller/1 -> out/1
  Constant1/1 -> PID Controller/2
  Constant2/1 -> PID Controller/3

== system model_constInput_IPC/Constant Input Selector/Cyclic Pitch Control/PI - D1 ==
  in : Inport
  Constant : Constant  Value=25
  DPI : Scope  NumInputPorts=3
  Discrete Derivative : simulink/Discrete/Discrete Derivative  gainval=1.0  ICPrevScaledInput=0.0  OutMin=[]  OutMax=[]  OutDataType=fixdt(1, 16)  OutScaling=2^-10  DoSatur=off
  Integrator : DiscreteIntegrator  IntegratorMethod=Integration: Backward Euler  gainval=1  InitialConditionSource=external  SampleTime=-1  UpperSaturationLimit=1.570796/(.008068634/9.5492966)/(1./(1.+pi/2/.109997))  LowerSaturationLimit=0  ICPrevOutput=DiscIntNeverNeededParam  ICPrevScaledInput=DiscIntNeverNeededParam
  Kd : Gain  Gain=simOpt.SLipc.DQ_Kd_1P
  Ki : Gain  Gain=simOpt.SLipc.DQ_Ki_1P
  Kp : Gain  Gain=simOpt.SLipc.DQ_Kp_1P
  Sum3 : Sum  Inputs=+++
  Wderiv : DiscreteFilter  Numerator=simOpt.SLipc.Wderiv.Numerator{1}  Denominator=simOpt.SLipc.Wderiv.Denominator{1}
  out : Outport  VectorParamsAs1DForOutWhenUnconnected=off
  wires:
  Wderiv/1 -> Kd/1
  Sum3/1 -> out/1
  Kp/1 -> DPI/2, Sum3/2  "P"
  Discrete Derivative/1 -> Sum3/1, DPI/1  "D"
  Kd/1 -> Discrete Derivative/1
  in/1 -> Ki/1, Wderiv/1, Kp/1
  Integrator/1 -> DPI/3, Sum3/3  "I"
  Ki/1 -> Integrator/1
  Constant/1 -> Integrator/2

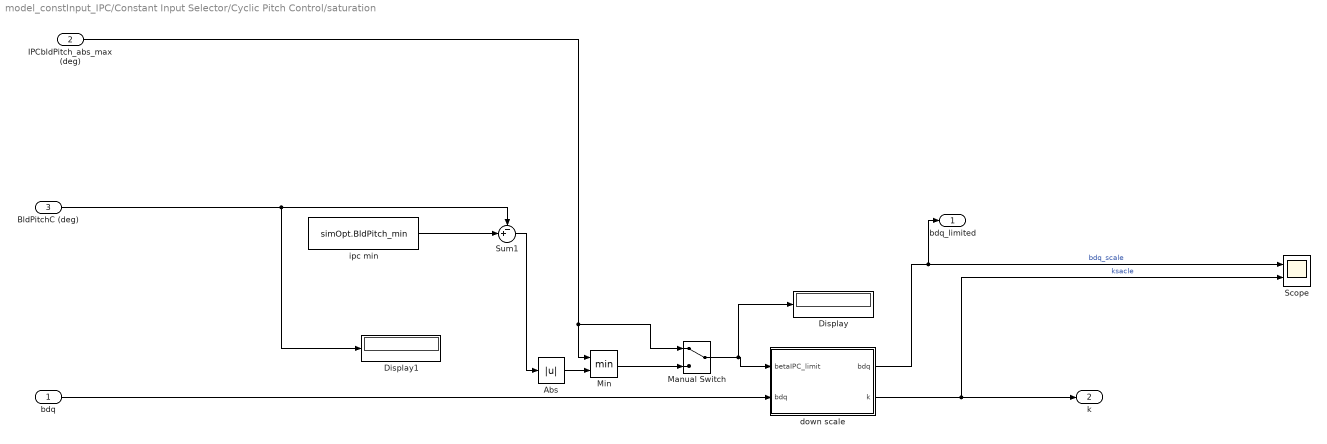
== system model_constInput_IPC/Constant Input Selector/Cyclic Pitch Control/saturation ==
  bdq : Inport
  IPCbldPitch_abs_max (deg) : Inport  Port=2
  BldPitchC (deg) : Inport  Port=3
  Abs : Abs
  Display : Display
  Display1 : Display
  Manual Switch : ManualSwitch
  Min : MinMax  Inputs=2
  Scope : Scope  NumInputPorts=2
  Sum1 : Sum  Inputs=-+|
  down scale : MATLAB Function  TreatAsAtomicUnit=on
  ipc min : Constant  Value=simOpt.BldPitch_min
  bdq_limited : Outport
  k : Outport  Port=2
  wires:
  ipc min/1 -> Sum1/2
  IPCbldPitch_abs_max (deg)/1 -> Manual Switch/1, Min/1
  bdq/1 -> down scale/2("bdq ")
  Sum1/1 -> Abs/1
  down scale/1(bdq) -> Scope/1, bdq_limited/1  "bdq_scale"
  down scale/2(k) -> Scope/2, k/1  "ksacle"
  BldPitchC (deg)/1 -> Display1/1, Sum1/1
  Abs/1 -> Min/2
  Min/1 -> Manual Switch/2
  Manual Switch/1 -> Display/1, down scale/1(betaIPC_limit)

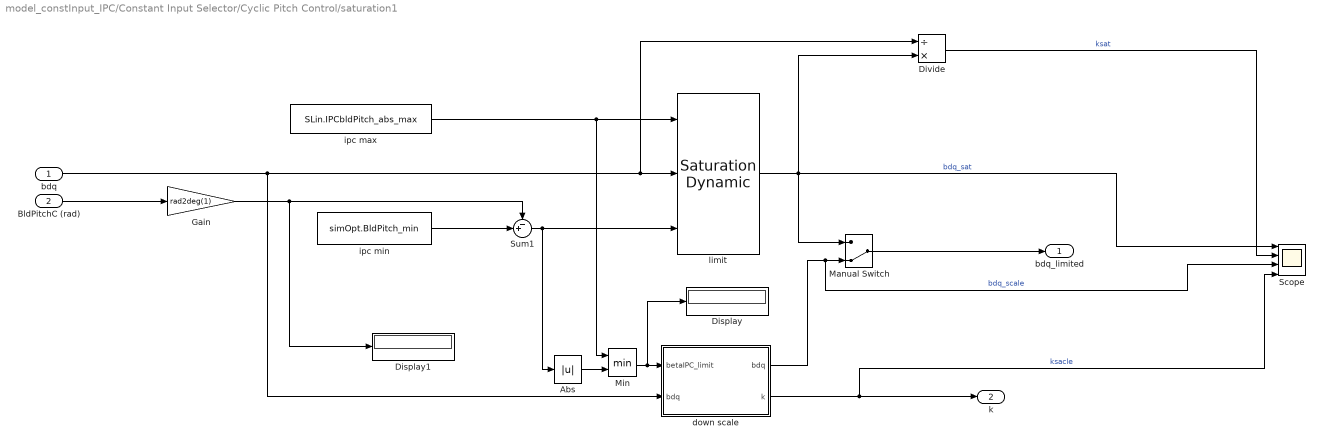
== system model_constInput_IPC/Constant Input Selector/Cyclic Pitch Control/saturation1 ==
  bdq : Inport
  BldPitchC (rad) : Inport  Port=2
  Abs : Abs
  Display : Display
  Display1 : Display
  Divide : Product  Inputs=/*
  Gain : Gain  Gain=rad2deg(1)
  Manual Switch : ManualSwitch  CurrentSetting=0
  Min : MinMax  Inputs=2
  Scope : Scope  NumInputPorts=4
  Sum1 : Sum  Inputs=-+|
  down scale : MATLAB Function  TreatAsAtomicUnit=on
  ipc max : Constant  Value=SLin.IPCbldPitch_abs_max
  ipc min : Constant  Value=simOpt.BldPitch_min
  limit : simulink/Discontinuities/Saturation Dynamic  OutMin=[]  OutMax=[]  OutDataTypeStr=Inherit: Same as second input  OutDataType=fixdt(1, 16)  OutScaling=2^-10  DoSatur=off
  bdq_limited : Outport
  k : Outport  Port=2
  wires:
  ipc min/1 -> Sum1/2
  ipc max/1 -> limit/1, Min/1
  limit/1 -> Scope/1, Manual Switch/1, Divide/2  "bdq_sat"
  bdq/1 -> down scale/2("bdq "), Divide/1, limit/2
  Manual Switch/1 -> bdq_limited/1
  BldPitchC (rad)/1 -> Gain/1
  Sum1/1 -> Abs/1, limit/3
  down scale/1(bdq) -> Scope/3, Manual Switch/2  "bdq_scale"
  down scale/2(k) -> k/1, Scope/4  "ksacle"
  Gain/1 -> Display1/1, Sum1/1
  Min/1 -> Display/1, down scale/1(betaIPC_limit)
  Divide/1 -> Scope/2  "ksat"
  Abs/1 -> Min/2

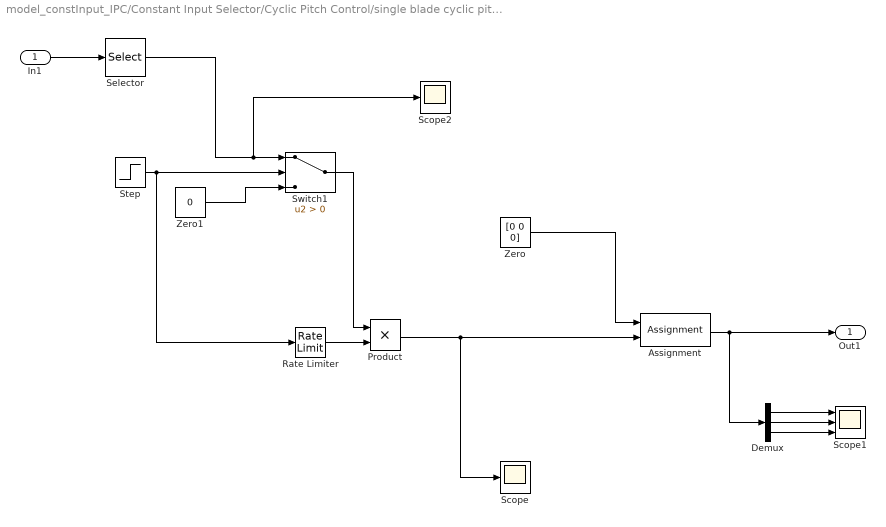
== system model_constInput_IPC/Constant Input Selector/Cyclic Pitch Control/single blade cyclic pitch ==
  In1 : Inport
  Assignment : Assignment  DiagnosticForDimensions=Warning  IndexOptions=Index vector (dialog)  Indices=1  OutputSizes=1
  Demux : Demux  Outputs=3
  Product : Product
  Rate Limiter : RateLimiter  RisingSlewLimit=0.1  SampleTimeMode=inherited
  Scope : Scope
  Scope1 : Scope  NumInputPorts=3
  Scope2 : Scope
  Selector : Selector  InputPortWidth=3  IndexOptions=Index vector (dialog)  Indices=[1]  OutputSizes=1
  Step : Step  Time=80  SampleTime=0
  Switch1 : Switch  Criteria=u2 > Threshold
  Zero : Constant  Value=[0 0 0]  OutDataTypeStr=Inherit: Inherit via back propagation
  Zero1 : Constant  Value=0  OutDataTypeStr=Inherit: Inherit via back propagation
  Out1 : Outport
  wires:
  Step/1 -> Rate Limiter/1, Switch1/2
  Zero1/1 -> Switch1/3
  Switch1/1 -> Product/1
  Product/1 -> Scope/1, Assignment/2
  Assignment/1 -> Demux/1, Out1/1
  Selector/1 -> Scope2/1, Switch1/1
  In1/1 -> Selector/1
  Rate Limiter/1 -> Product/2
  Demux/1 -> Scope1/1
  Demux/2 -> Scope1/2
  Demux/3 -> Scope1/3
  Zero/1 -> Assignment/1

== system model_constInput_IPC/Constant Input Selector/Cyclic Pitch Control/Filtering/Moving 3P Notch ==
  u : Inport
  RotSpeed (rad/s) : Inport  Port=2
  Gain : Gain  Gain=3
  Moving 3P Filt Manual : Subsystem  Commented=on
  Moving 3P Filter : cstblocks/Linear Parameter Varying/LPV System  sys=simOpt.SLipc.Wnotch3P  x0=0  uOffset=0  yOffset=0  xOffset=0  opEquilOption=on  dxOffset=0  sysFixedOption=Use the first model in state-space array  sysFixed=[]  AFixed=false  BFixed=false  CFixed=false  DFixed=false  uDelayFixed=false  yDelayFixed=false  iDelayFixed=false  IMethod=Linear  EMethod=Clip  IndexSearch=Binary search  IndexBegin=on  OutputX=off  OutputXdot=off  OutputLTI=off  OutputOP=off  DataType=double  SimMode=Interpreted execution  InitBufferSize=1024  FixedBuffer=off
      settings: SourceProductBaseCode=CT
  Rate Transition : RateTransition  Commented=on  OutPortSampleTime=DT
  y : Outport  VectorParamsAs1DForOutWhenUnconnected=off
  wires:
  Gain/1 -> Moving 3P Filter/2
  u/1 -> Moving 3P Filter/1
  Moving 3P Filter/1 -> y/1
  RotSpeed (rad/s)/1 -> Gain/1

== system model_constInput_IPC/Constant Input Selector/Cyclic Pitch Control/Filtering/Moving 6P Notch ==
  u : Inport
  RotSpeed (rad/s) : Inport  Port=2
  Gain : Gain  Gain=6
  Moving 6P Filter : cstblocks/Linear Parameter Varying/LPV System  sys=simOpt.SLipc.Wnotch6P  x0=0  uOffset=0  yOffset=0  xOffset=0  opEquilOption=on  dxOffset=0  sysFixedOption=Use the first model in state-space array  sysFixed=[]  AFixed=false  BFixed=false  CFixed=false  DFixed=false  uDelayFixed=false  yDelayFixed=false  iDelayFixed=false  IMethod=Linear  EMethod=Clip  IndexSearch=Binary search  IndexBegin=on  OutputX=off  OutputXdot=off  OutputLTI=off  OutputOP=off  DataType=double  SimMode=Interpreted execution  InitBufferSize=1024  FixedBuffer=off
      settings: SourceProductBaseCode=CT
  y : Outport  VectorParamsAs1DForOutWhenUnconnected=off
  wires:
  Gain/1 -> Moving 6P Filter/2
  u/1 -> Moving 6P Filter/1
  Moving 6P Filter/1 -> y/1
  RotSpeed (rad/s)/1 -> Gain/1

== system model_constInput_IPC/Constant Input Selector/Cyclic Pitch Control/Filtering/Moving Low Pass ==
  u : Inport
  RotSpeed (rad/s) : Inport  Port=2
  Gain : Gain  Gain=3
  Moving 6P Filter : cstblocks/Linear Parameter Varying/LPV System  sys=simOpt.SLipc.Wlowpass  x0=0  uOffset=0  yOffset=0  xOffset=0  opEquilOption=on  dxOffset=0  sysFixedOption=Use the first model in state-space array  sysFixed=[]  AFixed=false  BFixed=false  CFixed=false  DFixed=false  uDelayFixed=false  yDelayFixed=false  iDelayFixed=false  IMethod=Linear  EMethod=Clip  IndexSearch=Binary search  IndexBegin=on  OutputX=off  OutputXdot=off  OutputLTI=off  OutputOP=off  DataType=double  SimMode=Interpreted execution  InitBufferSize=1024  FixedBuffer=off
      settings: SourceProductBaseCode=CT
  y : Outport  VectorParamsAs1DForOutWhenUnconnected=off
  wires:
  Gain/1 -> Moving 6P Filter/2
  u/1 -> Moving 6P Filter/1
  Moving 6P Filter/1 -> y/1
  RotSpeed (rad/s)/1 -> Gain/1

== system model_constInput_IPC/Constant Input Selector/Cyclic Pitch Control/Filtering1/Moving 3P Notch ==
  u : Inport
  RotSpeed (rad/s) : Inport  Port=2
  Gain : Gain  Gain=3
  Moving 3P Filt Manual : Subsystem  Commented=on
  Moving 3P Filter : cstblocks/Linear Parameter Varying/LPV System  sys=simOpt.SLipc.Wnotch3P  x0=0  uOffset=0  yOffset=0  xOffset=0  opEquilOption=on  dxOffset=0  sysFixedOption=Use the first model in state-space array  sysFixed=[]  AFixed=false  BFixed=false  CFixed=false  DFixed=false  uDelayFixed=false  yDelayFixed=false  iDelayFixed=false  IMethod=Linear  EMethod=Clip  IndexSearch=Binary search  IndexBegin=on  OutputX=off  OutputXdot=off  OutputLTI=off  OutputOP=off  DataType=double  SimMode=Interpreted execution  InitBufferSize=1024  FixedBuffer=off
      settings: SourceProductBaseCode=CT
  Rate Transition : RateTransition  Commented=on  OutPortSampleTime=DT
  y : Outport  VectorParamsAs1DForOutWhenUnconnected=off
  wires:
  Gain/1 -> Moving 3P Filter/2
  u/1 -> Moving 3P Filter/1
  Moving 3P Filter/1 -> y/1
  RotSpeed (rad/s)/1 -> Gain/1

== system model_constInput_IPC/Constant Input Selector/Cyclic Pitch Control/Filtering1/Moving 6P Notch ==
  u : Inport
  RotSpeed (rad/s) : Inport  Port=2
  Gain : Gain  Gain=6
  Moving 6P Filter : cstblocks/Linear Parameter Varying/LPV System  sys=simOpt.SLipc.Wnotch6P  x0=0  uOffset=0  yOffset=0  xOffset=0  opEquilOption=on  dxOffset=0  sysFixedOption=Use the first model in state-space array  sysFixed=[]  AFixed=false  BFixed=false  CFixed=false  DFixed=false  uDelayFixed=false  yDelayFixed=false  iDelayFixed=false  IMethod=Linear  EMethod=Clip  IndexSearch=Binary search  IndexBegin=on  OutputX=off  OutputXdot=off  OutputLTI=off  OutputOP=off  DataType=double  SimMode=Interpreted execution  InitBufferSize=1024  FixedBuffer=off
      settings: SourceProductBaseCode=CT
  y : Outport  VectorParamsAs1DForOutWhenUnconnected=off
  wires:
  Gain/1 -> Moving 6P Filter/2
  u/1 -> Moving 6P Filter/1
  Moving 6P Filter/1 -> y/1
  RotSpeed (rad/s)/1 -> Gain/1

== system model_constInput_IPC/Constant Input Selector/Cyclic Pitch Control/Filtering1/Moving Low Pass ==
  u : Inport
  RotSpeed (rad/s) : Inport  Port=2
  Gain : Gain  Gain=3
  Moving 6P Filter : cstblocks/Linear Parameter Varying/LPV System  sys=simOpt.SLipc.Wlowpass  x0=0  uOffset=0  yOffset=0  xOffset=0  opEquilOption=on  dxOffset=0  sysFixedOption=Use the first model in state-space array  sysFixed=[]  AFixed=false  BFixed=false  CFixed=false  DFixed=false  uDelayFixed=false  yDelayFixed=false  iDelayFixed=false  IMethod=Linear  EMethod=Clip  IndexSearch=Binary search  IndexBegin=on  OutputX=off  OutputXdot=off  OutputLTI=off  OutputOP=off  DataType=double  SimMode=Interpreted execution  InitBufferSize=1024  FixedBuffer=off
      settings: SourceProductBaseCode=CT
  y : Outport  VectorParamsAs1DForOutWhenUnconnected=off
  wires:
  Gain/1 -> Moving 6P Filter/2
  u/1 -> Moving 6P Filter/1
  Moving 6P Filter/1 -> y/1
  RotSpeed (rad/s)/1 -> Gain/1

== system model_constInput_IPC/Constant Input Selector/Cyclic Pitch Control/Filtering/Moving 3P Notch/Moving 3P Filt Manual ==
  u : Inport
  RotSpeed (rad/s) : Inport  Port=2
  Den LPV : Subsystem
  Discrete Filter : DiscreteFilter  NumeratorSource=Input port  DenominatorSource=Input port  a0EqualsOne=on
      settings: InputPortMap=u0,p1,p3
  Num LPV : Subsystem
  Out1 : Outport  VectorParamsAs1DForOutWhenUnconnected=off
  wires:
  u/1 -> Discrete Filter/1
  Num LPV/1(b) -> Discrete Filter/2
  Discrete Filter/1 -> Out1/1
  RotSpeed (rad/s)/1 -> Den LPV/1(RotSpeed (rad/s)), Num LPV/1(RotSpeed (rad/s))
  Den LPV/1(a) -> Discrete Filter/3

== system model_constInput_IPC/Constant Input Selector/Cyclic Pitch Control/Filtering1/Moving 3P Notch/Moving 3P Filt Manual ==
  u : Inport
  RotSpeed (rad/s) : Inport  Port=2
  Den LPV : Subsystem
  Discrete Filter : DiscreteFilter  NumeratorSource=Input port  DenominatorSource=Input port  a0EqualsOne=on
      settings: InputPortMap=u0,p1,p3
  Num LPV : Subsystem
  Out1 : Outport  VectorParamsAs1DForOutWhenUnconnected=off
  wires:
  u/1 -> Discrete Filter/1
  Num LPV/1(b) -> Discrete Filter/2
  Discrete Filter/1 -> Out1/1
  RotSpeed (rad/s)/1 -> Den LPV/1(RotSpeed (rad/s)), Num LPV/1(RotSpeed (rad/s))
  Den LPV/1(a) -> Discrete Filter/3

== system model_constInput_IPC/Constant Input Selector/Cyclic Pitch Control/Filtering/Moving 3P Notch/Moving 3P Filt Manual/Den LPV ==
  RotSpeed (rad/s) : Inport
  1-D Lookup Table : Lookup_n-D  NumberOfTableDimensions=1  BreakpointsForDimension1=Parameter.Control.cIPC.PSM0_NF_3P.om_3P  BeginIndexSearchUsingPreviousIndexResult=on  Table=Parameter.Control.cIPC.PSM0_NF_3P.a_2  ExtrapMethod=Clip  InternalRulePriority=Speed  RndMeth=Simplest  InputSameDT=on
  1-D Lookup Table1 : Lookup_n-D  NumberOfTableDimensions=1  BreakpointsForDimension1=Parameter.Control.cIPC.PSM0_NF_3P.om_3P  BeginIndexSearchUsingPreviousIndexResult=on  Table=Parameter.Control.cIPC.PSM0_NF_3P.a_1  ExtrapMethod=Clip  InternalRulePriority=Speed  RndMeth=Simplest  InputSameDT=on
  1-D Lookup Table2 : Lookup_n-D  NumberOfTableDimensions=1  BreakpointsForDimension1=Parameter.Control.cIPC.PSM0_NF_3P.om_3P  BeginIndexSearchUsingPreviousIndexResult=on  Table=Parameter.Control.cIPC.PSM0_NF_3P.a_0  ExtrapMethod=Clip  InternalRulePriority=Speed  RndMeth=Simplest  InputSameDT=on
  Mux : Mux  Inputs=3
  a : Outport  VectorParamsAs1DForOutWhenUnconnected=off
  wires:
  1-D Lookup Table/1 -> Mux/1
  1-D Lookup Table1/1 -> Mux/2
  Mux/1 -> a/1
  RotSpeed (rad/s)/1 -> 1-D Lookup Table2/1, 1-D Lookup Table/1, 1-D Lookup Table1/1
  1-D Lookup Table2/1 -> Mux/3

== system model_constInput_IPC/Constant Input Selector/Cyclic Pitch Control/Filtering/Moving 3P Notch/Moving 3P Filt Manual/Num LPV ==
  RotSpeed (rad/s) : Inport
  1-D Lookup Table : Lookup_n-D  NumberOfTableDimensions=1  BreakpointsForDimension1=Parameter.Control.cIPC.PSM0_NF_3P.om_3P  BeginIndexSearchUsingPreviousIndexResult=on  Table=Parameter.Control.cIPC.PSM0_NF_3P.b_2  ExtrapMethod=Clip  InternalRulePriority=Speed  RndMeth=Simplest  InputSameDT=on
  1-D Lookup Table1 : Lookup_n-D  NumberOfTableDimensions=1  BreakpointsForDimension1=Parameter.Control.cIPC.PSM0_NF_3P.om_3P  BeginIndexSearchUsingPreviousIndexResult=on  Table=Parameter.Control.cIPC.PSM0_NF_3P.b_1  ExtrapMethod=Clip  InternalRulePriority=Speed  RndMeth=Simplest  InputSameDT=on
  1-D Lookup Table2 : Lookup_n-D  NumberOfTableDimensions=1  BreakpointsForDimension1=Parameter.Control.cIPC.PSM0_NF_3P.om_3P  BeginIndexSearchUsingPreviousIndexResult=on  Table=Parameter.Control.cIPC.PSM0_NF_3P.b_0  ExtrapMethod=Clip  InternalRulePriority=Speed  RndMeth=Simplest  InputSameDT=on
  Mux : Mux  Inputs=3
  b : Outport  VectorParamsAs1DForOutWhenUnconnected=off
  wires:
  1-D Lookup Table2/1 -> Mux/3
  RotSpeed (rad/s)/1 -> 1-D Lookup Table1/1, 1-D Lookup Table/1, 1-D Lookup Table2/1
  Mux/1 -> b/1
  1-D Lookup Table1/1 -> Mux/2
  1-D Lookup Table/1 -> Mux/1

== system model_constInput_IPC/Constant Input Selector/Cyclic Pitch Control/Filtering1/Moving 3P Notch/Moving 3P Filt Manual/Den LPV ==
  RotSpeed (rad/s) : Inport
  1-D Lookup Table : Lookup_n-D  NumberOfTableDimensions=1  BreakpointsForDimension1=Parameter.Control.cIPC.PSM0_NF_3P.om_3P  BeginIndexSearchUsingPreviousIndexResult=on  Table=Parameter.Control.cIPC.PSM0_NF_3P.a_2  ExtrapMethod=Clip  InternalRulePriority=Speed  RndMeth=Simplest  InputSameDT=on
  1-D Lookup Table1 : Lookup_n-D  NumberOfTableDimensions=1  BreakpointsForDimension1=Parameter.Control.cIPC.PSM0_NF_3P.om_3P  BeginIndexSearchUsingPreviousIndexResult=on  Table=Parameter.Control.cIPC.PSM0_NF_3P.a_1  ExtrapMethod=Clip  InternalRulePriority=Speed  RndMeth=Simplest  InputSameDT=on
  1-D Lookup Table2 : Lookup_n-D  NumberOfTableDimensions=1  BreakpointsForDimension1=Parameter.Control.cIPC.PSM0_NF_3P.om_3P  BeginIndexSearchUsingPreviousIndexResult=on  Table=Parameter.Control.cIPC.PSM0_NF_3P.a_0  ExtrapMethod=Clip  InternalRulePriority=Speed  RndMeth=Simplest  InputSameDT=on
  Mux : Mux  Inputs=3
  a : Outport  VectorParamsAs1DForOutWhenUnconnected=off
  wires:
  1-D Lookup Table/1 -> Mux/1
  1-D Lookup Table1/1 -> Mux/2
  Mux/1 -> a/1
  RotSpeed (rad/s)/1 -> 1-D Lookup Table2/1, 1-D Lookup Table/1, 1-D Lookup Table1/1
  1-D Lookup Table2/1 -> Mux/3

== system model_constInput_IPC/Constant Input Selector/Cyclic Pitch Control/Filtering1/Moving 3P Notch/Moving 3P Filt Manual/Num LPV ==
  RotSpeed (rad/s) : Inport
  1-D Lookup Table : Lookup_n-D  NumberOfTableDimensions=1  BreakpointsForDimension1=Parameter.Control.cIPC.PSM0_NF_3P.om_3P  BeginIndexSearchUsingPreviousIndexResult=on  Table=Parameter.Control.cIPC.PSM0_NF_3P.b_2  ExtrapMethod=Clip  InternalRulePriority=Speed  RndMeth=Simplest  InputSameDT=on
  1-D Lookup Table1 : Lookup_n-D  NumberOfTableDimensions=1  BreakpointsForDimension1=Parameter.Control.cIPC.PSM0_NF_3P.om_3P  BeginIndexSearchUsingPreviousIndexResult=on  Table=Parameter.Control.cIPC.PSM0_NF_3P.b_1  ExtrapMethod=Clip  InternalRulePriority=Speed  RndMeth=Simplest  InputSameDT=on
  1-D Lookup Table2 : Lookup_n-D  NumberOfTableDimensions=1  BreakpointsForDimension1=Parameter.Control.cIPC.PSM0_NF_3P.om_3P  BeginIndexSearchUsingPreviousIndexResult=on  Table=Parameter.Control.cIPC.PSM0_NF_3P.b_0  ExtrapMethod=Clip  InternalRulePriority=Speed  RndMeth=Simplest  InputSameDT=on
  Mux : Mux  Inputs=3
  b : Outport  VectorParamsAs1DForOutWhenUnconnected=off
  wires:
  1-D Lookup Table2/1 -> Mux/3
  RotSpeed (rad/s)/1 -> 1-D Lookup Table1/1, 1-D Lookup Table/1, 1-D Lookup Table2/1
  Mux/1 -> b/1
  1-D Lookup Table1/1 -> Mux/2
  1-D Lookup Table/1 -> Mux/1

== matlab function model_constInput_IPC/Constant Input Selector/Cyclic Pitch Control/saturation/down scale ==
  data: betaIPC_limit input; bdq input; bdq output; k output
function [bdq,k]  = bckMBC2(betaIPC_limit,bdq)
% This block supports the Embedded MATLAB subset.
% See the help menu for details.

d=bdq(1);
q=bdq(2);
psi_max=atan(q/d);
betaIPC_max=cos(psi_max)*d+sin(psi_max)*q; % largest deflection cmd due to IPC
k=min(abs(betaIPC_limit/betaIPC_max),1); % scaling factor
bdq=k*bdq;

== matlab function model_constInput_IPC/Constant Input Selector/Cyclic Pitch Control/MATLAB Function ==
  data: bdq input; beta output; Az input
function beta  = bckMBC2(bdq, Az)
% This block supports the Embedded MATLAB subset.
% See the help menu for details.

beta=[cosd(Az)       sind(Az); ...
      cosd(Az + 120) sind(Az + 120); ...
      cosd(Az + 240) sind(Az + 240)]*bdq(:);

== matlab function model_constInput_IPC/Constant Input Selector/Cyclic Pitch Control/saturation1/down scale ==
  data: betaIPC_limit input; bdq input; bdq output; k output
function [bdq,k]  = bckMBC2(betaIPC_limit,bdq)
% This block supports the Embedded MATLAB subset.
% See the help menu for details.

d=bdq(1);
q=bdq(2);
psi_max=atan(q/d);
betaIPC_max=cos(psi_max)*d+sin(psi_max)*q; % largest deflection cmd due to IPC
k=min(abs(betaIPC_limit/betaIPC_max),1); % scaling factor
bdq=k*bdq;

== matlab function model_constInput_IPC/Constant Input Selector/Cyclic Pitch Control/d-q transformation ==
  data: RootMyc input; M_tilt output; Az input; M_yaw output
function [M_tilt,M_yaw] = fwdMBC2(RootMyc, Az )
% This block supports the Embedded MATLAB subset.
% See the help menu for details.


%     My=RootMyb-mean(RootMyc); %remove mean
    My=RootMyc;
    M_tilt = (2/3).*[cosd(Az) cosd(Az+120) cosd(Az+240)]*My;
    M_yaw =  (2/3).*[sind(Az) sind(Az+120) sind(Az+240)]*My;
